simulink model "Simscape_Valve_Cylinder_8"  (R2014a)
settings: Solver=ode15s  StartTime=0.0  StopTime=10.0  RelTol=1e-3
PreLoadFcn:
  | leakage_area = 1e-9;
libraries: fl_lib x13, nesl_utility x3
Description:
  | Copyright 2014 The MathWorks, Inc.
settings Model: Creator=smiller  LastModifiedBy=smiller
settings DataIOCC: SignalLoggingSaveFormat=ModelDataLogs
settings OptimizationCC: ExpressionDepthLimit=2147483647  InitFltsAndDblsToZero=on
settings DebuggingCC: SaveWithParameterizedLinksMsg=none  UnderspecifiedInitializationDetection=Classic  FcnCallInpInsideContextMsg=UseLocalSettings  StateNameClashWarn=warning
settings GRTTargetCC: TargetFcnLib=ansi_tfl_tmw.mat  CombineOutputUpdateFcns=off  GRTInterface=on

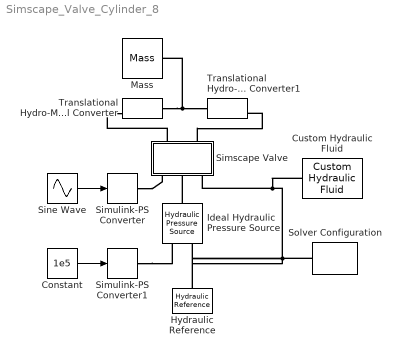
== system Simscape_Valve_Cylinder_8 ==
  Constant : Constant  Value=1e5
  Custom Hydraulic Fluid : fl_lib/Hydraulic/Hydraulic Utilities/Custom Hydraulic Fluid  density=850 kg/m^3  viscosity_kin=1.8e-05 m^2/s  bulk=8e+08 Pa  alpha=0.005  range_error=2
  Hydraulic Reference : fl_lib/Hydraulic/Hydraulic Elements/Hydraulic Reference
  Ideal Hydraulic Pressure Source : fl_lib/Hydraulic/Hydraulic Sources/Hydraulic Pressure Source
  Mass : fl_lib/Mechanical/Translational Elements/Mass  mass=1 kg  v_specify=on  v_priority=High  v=0 m/s  f_specify=off  f_priority=High  f=0 N
  Simscape Valve : Subsystem
  Simulink-PS Converter : nesl_utility/Simulink-PS Converter  PhysicalDomain=network_engine_domain  SubClassName=ps_input  LeftPortType=input  RightPortType=output  PseudoPeriodic=off  Frequencies=[]  NoiseDistribution=none  NoiseParameters=[]  Unit=m^2  AffineConversion=off  InputFiltering=off  SimscapeFilterOrder=1  InputFilterTimeConstant=.001  UdotUserProvided=0
  Simulink-PS Converter1 : nesl_utility/Simulink-PS Converter  PhysicalDomain=network_engine_domain  SubClassName=ps_input  LeftPortType=input  RightPortType=output  PseudoPeriodic=off  Frequencies=[]  NoiseDistribution=none  NoiseParameters=[]  Unit=Pa  AffineConversion=off  InputFiltering=off  SimscapeFilterOrder=1  InputFilterTimeConstant=.001  UdotUserProvided=0
  Sine Wave : Sin  Amplitude=1e-5  SampleTime=0
  Solver Configuration : nesl_utility/Solver Configuration  PhysicalDomain=network_engine_domain  SubClassName=solver  LeftPortType=input  RightPortType=generic  Accelerate=off  Tones=[]  Harmonics=[]  SimulateNoise=off  Profile=off  UseLocalSampling=off  EnableSwitchedLinearOptims=on  FrequencyDomain=off  UseCCode=off  RelTol=0.001  AbsTol=1e-06  MinStep=1e-09  ToWorkspace=off  DoDC=off  ResidualTolerance=1e-9  UseLocalSolver=off  LocalSolverChoice=NE_BACKWARD_EULER_ADVANCER  LocalSolverSampleTime=.001  DoFixedCost=off  MaxNonlinIter=12  MaxModeIter=2  LinearAlgebra=Sparse  DelaysMemoryBudget=1024  AutomaticFiltering=on  FilteringTimeConstant=0.001
  Translational Hydro-Mechanical Converter : fl_lib/Hydraulic/Hydraulic Elements/Translational Hydro-Mechanical Converter  area=5e-04 m^2  or=1  compressibility=0  init_pos=0 m  V_dead=1e-4 m^3  k_sh=1.4  initial_pressure=0 Pa
  Translational Hydro-Mechanical Converter1 : fl_lib/Hydraulic/Hydraulic Elements/Translational Hydro-Mechanical Converter  area=5e-04 m^2  or=2  compressibility=0  init_pos=0 m  V_dead=1e-4 m^3  k_sh=1.4  initial_pressure=0 Pa
  wires:
  Sine Wave/1 -> Simulink-PS Converter/1
  Constant/1 -> Simulink-PS Converter1/1
  connections:
  Simulink-PS Converter/RConn1 -- Simscape Valve/LConn1
  Solver Configuration/RConn1 -- Ideal Hydraulic Pressure Source/RConn2 -- Hydraulic Reference/LConn1 -- Simscape Valve/LConn3 -- Custom Hydraulic Fluid/RConn1
  Ideal Hydraulic Pressure Source/LConn1 -- Simscape Valve/LConn2
  Simulink-PS Converter1/RConn1 -- Ideal Hydraulic Pressure Source/RConn1
  Translational Hydro-Mechanical Converter/RConn1 -- Translational Hydro-Mechanical Converter1/RConn1 -- Mass/LConn1
  Simscape Valve/RConn2 -- Translational Hydro-Mechanical Converter1/LConn2
  Simscape Valve/RConn1 -- Translational Hydro-Mechanical Converter/LConn2

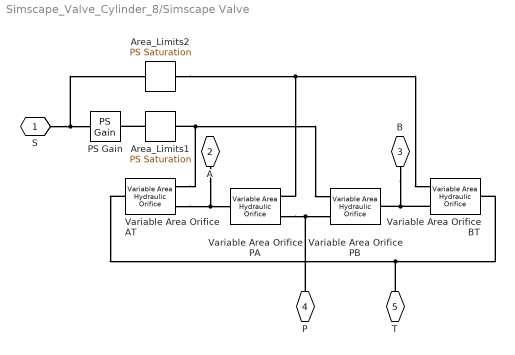
== system Simscape_Valve_Cylinder_8/Simscape Valve ==
  Area_Limits1 : fl_lib/Physical Signals/Nonlinear Operators/PS Saturation  upper_limit=1e-5 + leakage_area  lower_limit=leakage_area
  Area_Limits2 : fl_lib/Physical Signals/Nonlinear Operators/PS Saturation  upper_limit=1e-5 + leakage_area  lower_limit=leakage_area
  PS Gain : fl_lib/Physical Signals/Functions/PS Gain  gain=-1
  Variable Area Orifice AT : fl_lib/Hydraulic/Hydraulic Elements/Variable Area Hydraulic Orifice  C_d=0.7  Re_cr=12  min_area=1e-12 m^2  q_specify=off  q_priority=High  q=1 m^3/s  p_specify=off  p_priority=High  p=0 Pa
  Variable Area Orifice BT : fl_lib/Hydraulic/Hydraulic Elements/Variable Area Hydraulic Orifice  C_d=0.7  Re_cr=12  min_area=1e-12 m^2  q_specify=off  q_priority=High  q=1 m^3/s  p_specify=off  p_priority=High  p=0 Pa
  Variable Area Orifice PA : fl_lib/Hydraulic/Hydraulic Elements/Variable Area Hydraulic Orifice  C_d=0.7  Re_cr=12  min_area=1e-12 m^2  q_specify=off  q_priority=High  q=1 m^3/s  p_specify=off  p_priority=High  p=0 Pa
  Variable Area Orifice PB : fl_lib/Hydraulic/Hydraulic Elements/Variable Area Hydraulic Orifice  C_d=0.7  Re_cr=12  min_area=1e-12 m^2  q_specify=off  q_priority=High  q=1 m^3/s  p_specify=off  p_priority=High  p=0 Pa
  S : PMIOPort  Tag=PMCPort  Port=1  Side=Left
  A : PMIOPort  Tag=PMCPort  Port=2  Side=Right
  B : PMIOPort  Tag=PMCPort  Port=3  Side=Right
  P : PMIOPort  Tag=PMCPort  Port=4  Side=Left
  T : PMIOPort  Tag=PMCPort  Port=5  Side=Left
  connections:
  P/RConn1 -- Variable Area Orifice PA/LConn2 -- Variable Area Orifice PB/LConn2
  B/RConn1 -- Variable Area Orifice BT/LConn2 -- Variable Area Orifice PB/RConn1
  A/RConn1 -- Variable Area Orifice AT/LConn2 -- Variable Area Orifice PA/RConn1
  Variable Area Orifice AT/RConn1 -- T/RConn1 -- Variable Area Orifice BT/RConn1
  S/RConn1 -- PS Gain/LConn1 -- Area_Limits2/LConn1
  Variable Area Orifice PB/LConn1 -- Variable Area Orifice AT/LConn1 -- Area_Limits1/RConn1
  Area_Limits1/LConn1 -- PS Gain/RConn1
  Area_Limits2/RConn1 -- Variable Area Orifice BT/LConn1 -- Variable Area Orifice PA/LConn1
